simulink model "Hierarchy1"  (Simulink 5.0)
settings: Solver=ode45  StartTime=0.0  StopTime=10.0  RelTol=1e-3
settings Model: Creator=scaife  LastModifiedBy=scaife  ExtModeAutoUpdateStatusClock=off

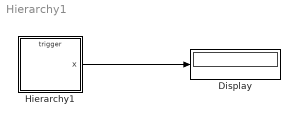
== system Hierarchy1 ==
  Display : Display
  Hierarchy1 : Stateflow chart
  wires:
  Hierarchy1/1(x) -> Display/1

== stateflow chart Hierarchy1 ==
  state TOP/ en:x+=1000000; ex:x=0;
    state N1/
      en:x+=10000;
      ex:x-=10000;
      state A/
        en: x+=10;
      state B/
        en: x-=10;
      (default) -> A
      A -> B : S{x+=1;}
      B -> A : R{x-=1;}
    state N2/
      en:x+=100000;
      ex:x-=100000;
      state C/
        en: x+=1000;
      state D/
        en: x-=1000;
      (default) -> C
      C -> D : S{x+=100;}
      D -> C : R{x-=100;}
    (default) -> N1
    N1 -> N2 : T
    N2 -> N1 : T
  (default) -> TOP/ en:x+=1000000; ex:x=0;
  data: x output double
  events: S input EITHER_EDGE_EVENT; R input EITHER_EDGE_EVENT; T input EITHER_EDGE_EVENT
